simulink model "ex01"  (R2022b)
settings: Solver=VariableStepAuto  StartTime=0.0  StopTime=50  RelTol=1e-3
settings Model: Creator=ACER  LastModifiedBy=ACER

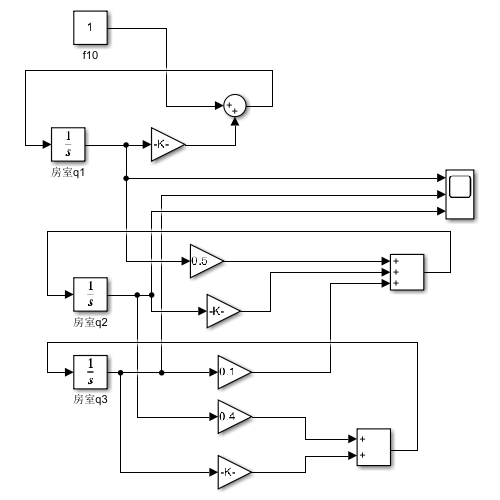
[thumbnail: Simulink's stored preview of the top-level diagram]
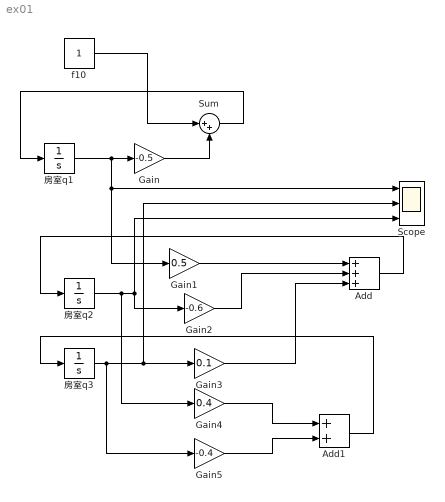
== system ex01 ==
  Add : Sum  Inputs=+++
  Add1 : Sum
  Gain : Gain  Gain=-0.5
  Gain1 : Gain  Gain=0.5
  Gain2 : Gain  Gain=-0.6
  Gain3 : Gain  Gain=0.1
  Gain4 : Gain  Gain=0.4
  Gain5 : Gain  Gain=-0.4
  Scope : Scope  NumInputPorts=3
  Sum : Sum  Inputs=|++
  f10 : Constant
  房室q1 : Integrator  Tag=房室q1  InitialCondition=1
  房室q2 : Integrator  Tag=房室q2  InitialCondition=10
  房室q3 : Integrator  Tag=房室q3
  wires:
  房室q1/1 -> Gain1/1, Scope/1, Gain/1
  Gain/1 -> Sum/2
  f10/1 -> Sum/1
  Sum/1 -> 房室q1/1
  房室q2/1 -> Gain4/1, Scope/3, Gain2/1
  房室q3/1 -> Gain5/1, Scope/2, Gain3/1
  Gain1/1 -> Add/1
  Gain2/1 -> Add/2
  Gain3/1 -> Add/3
  Add/1 -> 房室q2/1
  Gain4/1 -> Add1/1
  Gain5/1 -> Add1/2
  Add1/1 -> 房室q3/1
